simulink model "HEV_Simu_V1_1_RT"  (R2018a)
settings: Solver=ode23s  StartTime=0.0  StopTime=660  FixedStep=0.001  EnableMultiTasking=on
PreLoadFcn:
  | HevSimuVccWs_V1_PreLoad
StartFcn:
  | tic
StopFcn:
  | toc
  | disp(['実時間の' num2str(max(tout)/toc) '倍速'])
model workspace (MAT data in the model file):
  Var = 0
undefined symbols (not defined in the file or in its folder): canChannel
libraries: canmsglib x55, canlib x35, simulink x2, sldrtlib x1
(part 1 of 4)
Description:
  | Ver1 ：
settings Model: SimulationMode=accelerator  Creator=1442442  LastModifiedBy=E00026
settings SolverCC: MaxOrder=2  ZeroCrossControl=DisableAll
settings DataIOCC: SaveFormat=Array  SaveOutput=off  SignalLogging=off  DSMLogging=off
settings OptimizationCC: ExpressionDepthLimit=2147483647  EfficientMapNaN2IntZero=off  LifeSpan=inf
settings DebuggingCC: AlgebraicLoopMsg=error  UnderspecifiedInitializationDetection=Classic  MergeDetectMultiDrivingBlocksExec=none  FcnCallInpInsideContextMsg=warning  StateNameClashWarn=warning  SFUnexpectedBacktrackingDiag=warning  SFNoUnconditionalDefaultTransitionDiag=warning  SFExecutionAtInitializationDiag=none
settings HardwareCC: ProdBitPerPointer=32  ProdBitPerSizeT=32  ProdBitPerPtrDiffT=32  ProdLargestAtomicFloat=None  ProdIntDivRoundTo=Undefined  ProdEndianess=Unspecified  ProdWordSize=32  ProdHWDeviceType=32-bit Generic  TargetBitPerPointer=64  TargetBitPerSizeT=64  TargetBitPerPtrDiffT=64  TargetLongLongMode=on  TargetIntDivRoundTo=Zero  TargetEndianess=LittleEndian  TargetWordSize=64  TargetHWDeviceType=MATLAB Host  ProdEqTarget=off
settings ModelReferenceCC: PropagateSignalLabelsOutOfModel=off
settings CodeAppCC: MaxIdLength=128
settings GRTTargetCC: TargetLangStandard=C89/C90 (ANSI)  CombineOutputUpdateFcns=off  GRTInterface=on
settings ConfigComp: CovMetricSettings=dw  CovHtmlReporting=on  CovSaveCumulativeToWorkspaceVar=on  CovSaveSingleToWorkspaceVar=on  CovExternalEMLEnable=off  CovSFcnEnable=off
settings SimscapeCC: SimscapeNormalizeSystem=off  SimscapeLogSimulationStatistics=on  SimscapeLogOpenViewer=on  SimscapeLogLimitData=off

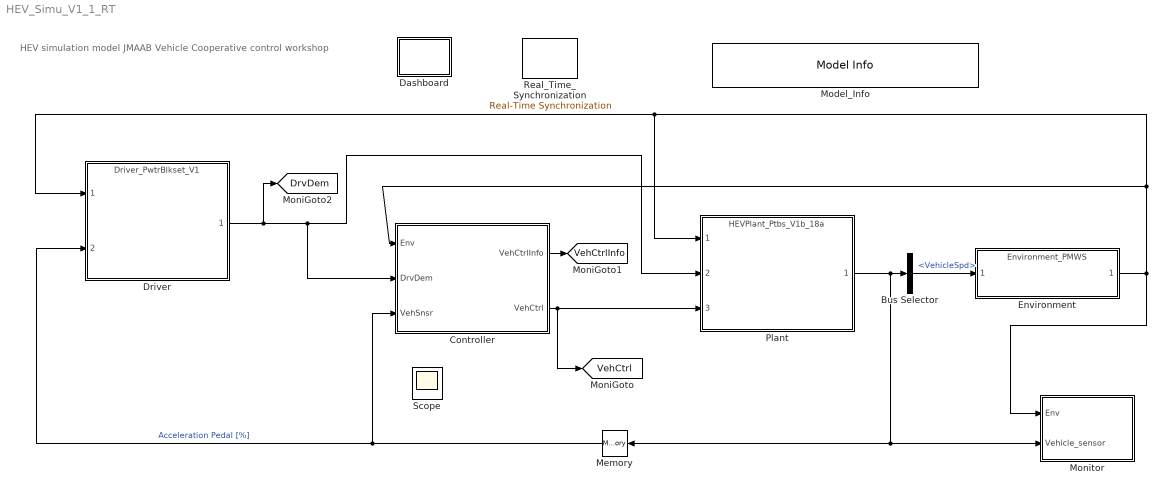
== system HEV_Simu_V1_1_RT ==
  note: HEV simulation model
      | JMAAB Vehicle Cooperative control workshop
  Bus Selector : BusSelector  OutputSignals=Brake_sensor.VehicleSpd
  Controller : Subsystem  Variant=on  PropagateVariantConditions=on
  Dashboard : Subsystem
  Driver : ModelReference  ModelNameDialog=Driver_PwtrBlkset_V1.slx  SimulationMode=Normal  ModelReferenceVersion=1.1301
  Environment : ModelReference  ModelNameDialog=Environment_PMWS.slx  SimulationMode=Normal  ModelReferenceVersion=1.1285
  Memory : Memory
  Model_Info : simulink/Model-Wide Utilities/Model Info  Frame=on  DisplayStringWithTags=|  HorizontalTextAlignment=Left  LeftAlignmentValue=0.02
      | Version  %<ModelVersion>
      | LastModifided by %<LastModifiedBy>  Date %<LastModificationDate>
      | Description  %<Description>
  Monitor : Subsystem
  Plant : ModelReference  ModelNameDialog=HEVPlant_Ptbs_V1b_18a.slx  SimulationMode=Normal  ModelReferenceVersion=1.1342
  Real_Time_Synchronization : sldrtlib/Real-Time Synchronization  SampleTime=0.01  MaxMissedTicks=100  ShowMissedTicks=off  YieldWhenWaiting=off
      settings: AttributesFormatString=<MaxMissedTicks = %<MaxMissedTicks>>
  Scope : Scope
  tag scope: DrvDem=global, VehCtrl=global, VehCtrlInfo=global
  wires:
  Bus Selector/1 -> Environment/1  "<VehicleSpd>"
  Memory/1 -> Driver/2, Controller/3(VehSnsr)  "Acceleration Pedal [%]"
  Plant/1 -> Monitor/2(Vehicle_sensor), Memory/1, Bus Selector/1
  Driver/1 -> Controller/2("DrvDem "), Plant/2, [DrvDem]
  Environment/1 -> Plant/1, Driver/1, Controller/1("Env "), Monitor/1(Env)
  Controller/1(" VehCtrlInfo") -> [VehCtrlInfo]
  Controller/2(" VehCtrl") -> Plant/3, [VehCtrl]

== system HEV_Simu_V1_1_RT/Controller ==
  "Env " : Inport
  "DrvDem " : Inport  Port=2
  VehSnsr : Inport  Port=3
  CtrlStrct_SmplCAN.slx : ModelReference  ModelNameDialog=CtrlStrct_SmplCAN.slx  SimulationMode=Normal  VariantControl=VarObj_CtrlStruct_CAN_Simpl  ModelReferenceVersion=0.1.90
  CtrlStrct_SmplCAN_Intg.slx : ModelReference  ModelNameDialog=CtrlStrct_SmplCAN_Intg.slx  SimulationMode=Normal  VariantControl=(default)  ModelReferenceVersion=0.1.68
  CtrlStrct_SmplCAN_TW.slx : ModelReference  ModelNameDialog=CtrlStrct_SmplCAN_TW.slx  SimulationMode=Normal  VariantControl=VarObj_CtrlStruct_CAN_Simpl_TW  ModelReferenceVersion=0.1.89
  CtrlStrct_VNT_Level_1 : ModelReference  ModelNameDialog=CtrlStrct_VNT_Level1_TW.slx  SimulationMode=Normal  VariantControl=VarObj_CtrlStruct_CAN_VNT_Level_1  ModelReferenceVersion=0.1.98
  CtrlStrct_VNT_Level_2 : Subsystem  TreatAsAtomicUnit=on  VariantControl=VarObj_CtrlStruct_CAN_VNT_Level_2
  " VehCtrlInfo" : Outport
  " VehCtrl" : Outport  Port=2

== system HEV_Simu_V1_1_RT/Dashboard ==
  note: Battery SOC
  note: Brake Pedal
  note: Accel Pedal
  note: Engine Speed
  note: Vehicle Speed
  note: Engine Torque Dem
  note: Clutch Dem
  note: Motor Torque Dem
  Dashboard Scope : Subsystem  DialogController=hmiCreateDDGDialog  IsWebBlock=on  mask(MWDashboardBlock){webBlockId=ed88d156-d389-420b-ac55-88fe2db30599, webBlockType=sdiscope, ShowInitialText=on, HMISrcModelName=HEV_Simu_V1_1_RT}
      mask prompts: webBlockId "WebBlock Id"; webBlockType "WebBlock Type"; HMISrcModelName "Source Model"
      mask help: SimulinkHMI:dialogs:HMIScopeDialogDesc
      mask Help: helpview([docroot '/mapfiles/simulink.map'], 'hmi_scope')
      mask Display:
      | if strcmp(get_param(bdroot(gcb),'BlockDiagramType'), 'library')
      |     image([(matlabroot) '/toolbox/simulink/hmi/icons/DashboardScope.png']);
      | end
  Gauge : Subsystem  DialogController=hmiCreateDDGDialog  IsWebBlock=on  mask(MWDashboardBlock){webBlockId=63f936d2-1b71-4121-bdb3-6f8d7f4bf67f, webBlockType=circulargauge, ShowInLibBrowser=on, ShowInitialText=on, HMISrcModelName=HEV_Simu_V1_1_RT}
      mask prompts: webBlockId "WebBlock Id"; webBlockType "WebBlock Type"; HMISrcModelName "Source Model"
      mask help: SimulinkHMI:dialogs:CircularGaugeDialogDesc
      mask Help: helpview([docroot '/mapfiles/simulink.map'], 'hmi_gauge')
      mask Display:
      | if strcmp(get_param(bdroot(gcb),'BlockDiagramType'), 'library')
      |     image([(matlabroot) '/toolbox/simulink/hmi/icons/CircularGauge.png']);
      | end
  Gauge1 : Subsystem  DialogController=hmiCreateDDGDialog  IsWebBlock=on  mask(MWDashboardBlock){webBlockId=f9ab9f1f-3ce6-4036-8e0e-91baa74d8dba, webBlockType=circulargauge, ShowInLibBrowser=on, ShowInitialText=on, HMISrcModelName=HEV_Simu_V1_1_RT}
      mask prompts: webBlockId "WebBlock Id"; webBlockType "WebBlock Type"; HMISrcModelName "Source Model"
      mask help: SimulinkHMI:dialogs:CircularGaugeDialogDesc
      mask Help: helpview([docroot '/mapfiles/simulink.map'], 'hmi_gauge')
      mask Display:
      | if strcmp(get_param(bdroot(gcb),'BlockDiagramType'), 'library')
      |     image([(matlabroot) '/toolbox/simulink/hmi/icons/CircularGauge.png']);
      | end
  Linear Gauge : Subsystem  DialogController=hmiCreateDDGDialog  IsWebBlock=on  mask(MWDashboardBlock){webBlockId=d39eeb4b-9fab-4e2b-bb63-54dd45bd1f7c, webBlockType=lineargauge, ShowInLibBrowser=on, ShowInitialText=on, HMISrcModelName=HEV_Simu_V1_1_RT}
      mask prompts: webBlockId "WebBlock Id"; webBlockType "WebBlock Type"; HMISrcModelName "Source Model"
      mask help: SimulinkHMI:dialogs:LinearGaugeDialogDesc
      mask Help: helpview([docroot '/mapfiles/simulink.map'], 'hmi_linear_gauge')
      mask Display:
      | if strcmp(get_param(bdroot(gcb),'BlockDiagramType'), 'library')
      |     image([(matlabroot) '/toolbox/simulink/hmi/icons/LinearGauge.png']);
      | end
  Linear Gauge1 : Subsystem  DialogController=hmiCreateDDGDialog  IsWebBlock=on  mask(MWDashboardBlock){webBlockId=fb227460-5497-40ec-922f-134b3e225288, webBlockType=lineargauge, ShowInLibBrowser=on, ShowInitialText=on, HMISrcModelName=HEV_Simu_V1_1_RT}
      mask prompts: webBlockId "WebBlock Id"; webBlockType "WebBlock Type"; HMISrcModelName "Source Model"
      mask help: SimulinkHMI:dialogs:LinearGaugeDialogDesc
      mask Help: helpview([docroot '/mapfiles/simulink.map'], 'hmi_linear_gauge')
      mask Display:
      | if strcmp(get_param(bdroot(gcb),'BlockDiagramType'), 'library')
      |     image([(matlabroot) '/toolbox/simulink/hmi/icons/LinearGauge.png']);
      | end
  Linear Gauge2 : Subsystem  DialogController=hmiCreateDDGDialog  IsWebBlock=on  mask(MWDashboardBlock){webBlockId=1d5b4a74-8e32-404d-8aff-08484f192aeb, webBlockType=lineargauge, ShowInLibBrowser=on, ShowInitialText=on, HMISrcModelName=HEV_Simu_V1_1_RT}
      mask prompts: webBlockId "WebBlock Id"; webBlockType "WebBlock Type"; HMISrcModelName "Source Model"
      mask help: SimulinkHMI:dialogs:LinearGaugeDialogDesc
      mask Help: helpview([docroot '/mapfiles/simulink.map'], 'hmi_linear_gauge')
      mask Display:
      | if strcmp(get_param(bdroot(gcb),'BlockDiagramType'), 'library')
      |     image([(matlabroot) '/toolbox/simulink/hmi/icons/LinearGauge.png']);
      | end
  Linear Gauge3 : Subsystem  DialogController=hmiCreateDDGDialog  IsWebBlock=on  mask(MWDashboardBlock){webBlockId=8d479cc7-cf22-4f0e-9a8d-8e93dc3b7c1a, webBlockType=lineargauge, ShowInLibBrowser=on, ShowInitialText=on, HMISrcModelName=HEV_Simu_V1_1_RT}
      mask prompts: webBlockId "WebBlock Id"; webBlockType "WebBlock Type"; HMISrcModelName "Source Model"
      mask help: SimulinkHMI:dialogs:LinearGaugeDialogDesc
      mask Help: helpview([docroot '/mapfiles/simulink.map'], 'hmi_linear_gauge')
      mask Display:
      | if strcmp(get_param(bdroot(gcb),'BlockDiagramType'), 'library')
      |     image([(matlabroot) '/toolbox/simulink/hmi/icons/LinearGauge.png']);
      | end
  Linear Gauge4 : Subsystem  DialogController=hmiCreateDDGDialog  IsWebBlock=on  mask(MWDashboardBlock){webBlockId=595c5480-ce82-49fb-a87f-a471381cfd80, webBlockType=lineargauge, ShowInLibBrowser=on, ShowInitialText=on, HMISrcModelName=HEV_Simu_V1_1_RT}
      mask prompts: webBlockId "WebBlock Id"; webBlockType "WebBlock Type"; HMISrcModelName "Source Model"
      mask help: SimulinkHMI:dialogs:LinearGaugeDialogDesc
      mask Help: helpview([docroot '/mapfiles/simulink.map'], 'hmi_linear_gauge')
      mask Display:
      | if strcmp(get_param(bdroot(gcb),'BlockDiagramType'), 'library')
      |     image([(matlabroot) '/toolbox/simulink/hmi/icons/LinearGauge.png']);
      | end
  Linear Gauge5 : Subsystem  DialogController=hmiCreateDDGDialog  IsWebBlock=on  mask(MWDashboardBlock){webBlockId=43b93f51-ee21-4470-88be-b6fb93d81e08, webBlockType=lineargauge, ShowInLibBrowser=on, ShowInitialText=on, HMISrcModelName=HEV_Simu_V1_1_RT}
      mask prompts: webBlockId "WebBlock Id"; webBlockType "WebBlock Type"; HMISrcModelName "Source Model"
      mask help: SimulinkHMI:dialogs:LinearGaugeDialogDesc
      mask Help: helpview([docroot '/mapfiles/simulink.map'], 'hmi_linear_gauge')
      mask Display:
      | if strcmp(get_param(bdroot(gcb),'BlockDiagramType'), 'library')
      |     image([(matlabroot) '/toolbox/simulink/hmi/icons/LinearGauge.png']);
      | end

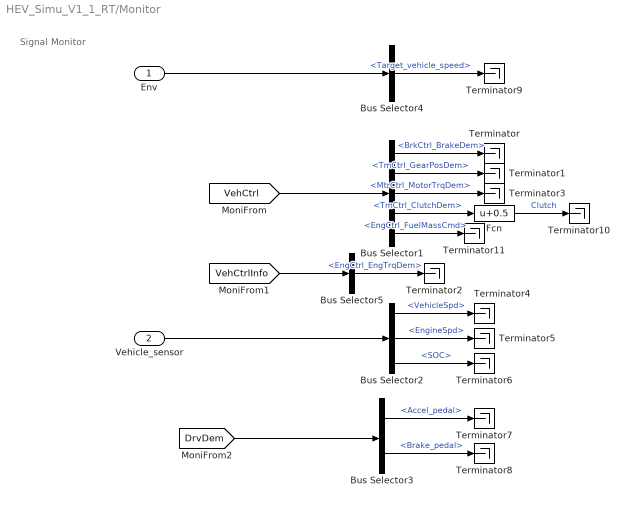
== system HEV_Simu_V1_1_RT/Monitor ==
  note: Signal Monitor
  Env : Inport
  Vehicle_sensor : Inport  Port=2
  Bus Selector1 : BusSelector  OutputSignals=BrakeCtrl.BrkCtrl_BrakeDem,TransmCtrl.TmCtrl_GearPosDem,MotorCtrl.MtrCtrl_MotorTrqDem,TransmCtrl.TmCtrl_ClutchDem,EngineCtrl.EngCtrl_FuelMassCmd
  Bus Selector2 : BusSelector  OutputSignals=Brake_sensor.VehicleSpd,Engine_sensor.EngineSpd,Battery_sensor.SOC
  Bus Selector3 : BusSelector  OutputSignals=Accel_pedal,Brake_pedal
  Bus Selector4 : BusSelector  OutputSignals=Target_vehicle_speed
  Bus Selector5 : BusSelector  OutputSignals=EngineCtrl_Info.EngCtrl_EngTrqDem
  Fcn : Fcn  Expr=u+0.5
  Terminator{,1..11} (12 alike) : Terminator
  wires:
  [VehCtrl] -> Bus Selector1/1
  Vehicle_sensor/1 -> Bus Selector2/1
  Bus Selector1/2 -> Terminator1/1  "<TmCtrl_GearPosDem>"
  Bus Selector1/3 -> Terminator3/1  "<MtrCtrl_MotorTrqDem>"
  Bus Selector2/1 -> Terminator4/1  "<VehicleSpd>"
  Bus Selector2/2 -> Terminator5/1  "<EngineSpd>"
  Bus Selector2/3 -> Terminator6/1  "<SOC>"
  Bus Selector1/1 -> Terminator/1  "<BrkCtrl_BrakeDem>"
  [DrvDem] -> Bus Selector3/1
  Bus Selector3/1 -> Terminator7/1  "<Accel_pedal>"
  Bus Selector3/2 -> Terminator8/1  "<Brake_pedal>"
  Env/1 -> Bus Selector4/1
  Bus Selector4/1 -> Terminator9/1  "<Target_vehicle_speed>"
  [VehCtrlInfo] -> Bus Selector5/1
  Bus Selector5/1 -> Terminator2/1  "<EngCtrl_EngTrqDem>"
  Bus Selector1/4 -> Fcn/1  "<TmCtrl_ClutchDem>"
  Fcn/1 -> Terminator10/1  "Clutch"
  Bus Selector1/5 -> Terminator11/1  "<EngCtrl_FuelMassCmd>"

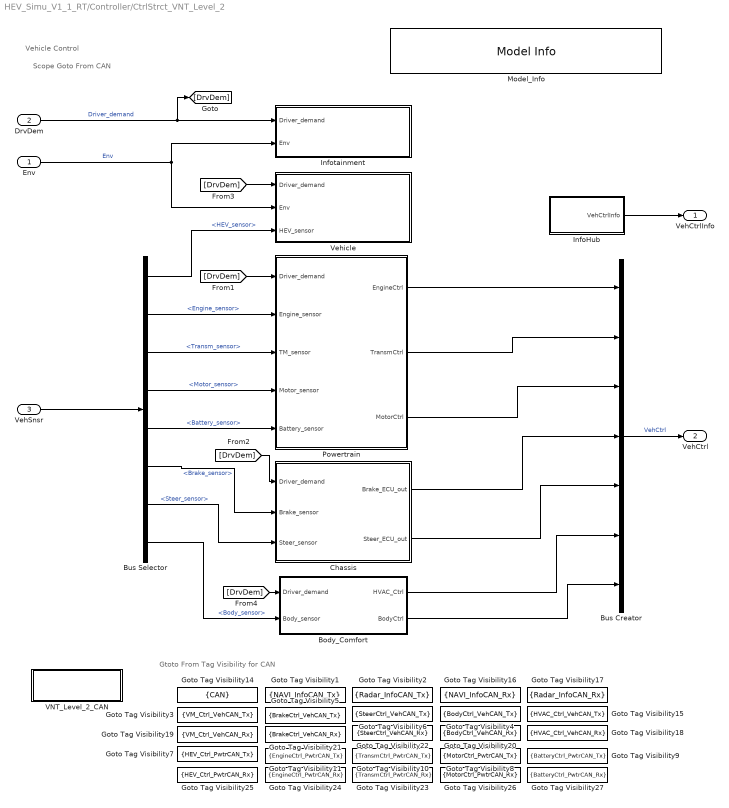
== system HEV_Simu_V1_1_RT/Controller/CtrlStrct_VNT_Level_2 ==
  note: Vehicle Control
  note: Gtoto From Tag Visibility for CAN
  note: Scope Goto From CAN
  Env : Inport  OutDataTypeStr=Bus: Environment_Bus
      settings: AttributesFormatString=<%<OutDataTypeStr>>
  DrvDem : Inport  Port=2  OutDataTypeStr=Bus: Driver_demand_Bus
      settings: AttributesFormatString=%<OutDataTypeStr>
  VehSnsr : Inport  Port=3  OutDataTypeStr=Bus: Vehicle_sensor_Bus
      settings: AttributesFormatString=<%<OutDataTypeStr>>
  Body_Comfort : Subsystem
  Bus Creator : BusCreator  Inputs=7  OutDataTypeStr=Bus: Ctrl_intg_Bus
      settings: AttributesFormatString=%<OutDataTypeStr>
  Bus Selector : BusSelector  OutputSignals=HEV_sensor,Engine_sensor,Transm_sensor,Motor_sensor,Battery_sensor,Brake_sensor,Steer_sensor,Body_sensor
  Chassis : Subsystem
  Goto Tag Visibility1 : GotoTagVisibility  GotoTag=NAVI_InfoCAN_Tx
  Goto Tag Visibility10 : GotoTagVisibility  GotoTag=TransmCtrl_PwtrCAN_Tx
  Goto Tag Visibility11 : GotoTagVisibility  GotoTag=EngineCtrl_PwtrCAN_Tx
  Goto Tag Visibility14 : GotoTagVisibility  GotoTag=CAN
  Goto Tag Visibility15 : GotoTagVisibility  GotoTag=HVAC_Ctrl_VehCAN_Tx
  Goto Tag Visibility16 : GotoTagVisibility  GotoTag=NAVI_InfoCAN_Rx
  Goto Tag Visibility17 : GotoTagVisibility  GotoTag=Radar_InfoCAN_Rx
  Goto Tag Visibility18 : GotoTagVisibility  GotoTag=HVAC_Ctrl_VehCAN_Rx
  Goto Tag Visibility19 : GotoTagVisibility  GotoTag=VM_Ctrl_VehCAN_Rx
  Goto Tag Visibility2 : GotoTagVisibility  GotoTag=Radar_InfoCAN_Tx
  Goto Tag Visibility20 : GotoTagVisibility  GotoTag=BodyCtrl_VehCAN_Rx
  Goto Tag Visibility21 : GotoTagVisibility  GotoTag=BrakeCtrl_VehCAN_Rx
  Goto Tag Visibility22 : GotoTagVisibility  GotoTag=SteerCtrl_VehCAN_Rx
  Goto Tag Visibility23 : GotoTagVisibility  GotoTag=TransmCtrl_PwtrCAN_Rx
  Goto Tag Visibility24 : GotoTagVisibility  GotoTag=EngineCtrl_PwtrCAN_Rx
  Goto Tag Visibility25 : GotoTagVisibility  GotoTag=HEV_Ctrl_PwtrCAN_Rx
  Goto Tag Visibility26 : GotoTagVisibility  GotoTag=MotorCtrl_PwtrCAN_Rx
  Goto Tag Visibility27 : GotoTagVisibility  GotoTag=BatteryCtrl_PwtrCAN_Rx
  Goto Tag Visibility3 : GotoTagVisibility  GotoTag=VM_Ctrl_VehCAN_Tx
  Goto Tag Visibility4 : GotoTagVisibility  GotoTag=BodyCtrl_VehCAN_Tx
  Goto Tag Visibility5 : GotoTagVisibility  GotoTag=BrakeCtrl_VehCAN_Tx
  Goto Tag Visibility6 : GotoTagVisibility  GotoTag=SteerCtrl_VehCAN_Tx
  Goto Tag Visibility7 : GotoTagVisibility  GotoTag=HEV_Ctrl_PwtrCAN_Tx
  Goto Tag Visibility8 : GotoTagVisibility  GotoTag=MotorCtrl_PwtrCAN_Tx
  Goto Tag Visibility9 : GotoTagVisibility  GotoTag=BatteryCtrl_PwtrCAN_Tx
  InfoHub : Subsystem
  Infotainment : Subsystem
  Model_Info : simulink/Model-Wide Utilities/Model Info  Frame=on  DisplayStringWithTags=|  HorizontalTextAlignment=Left  LeftAlignmentValue=0.02
      | Version  %<ModelVersion>
      | LastModifided by %<LastModifiedBy>  Date %<LastModificationDate>
      | Description  %<Description>
  Powertrain : Subsystem
  VNT_Level_2_CAN : Subsystem  VariantControl=VarObj_CanType_VNT_simu
  Vehicle : Subsystem
  VehCtrlInfo : Outport  OutDataTypeStr=Bus: IntgCtrl_Info_Bus
      settings: AttributesFormatString=<%<OutDataTypeStr>>
  VehCtrl : Outport  Port=2  OutDataTypeStr=Bus: Ctrl_intg_Bus
      settings: AttributesFormatString=<%<OutDataTypeStr>>
  wires:
  Chassis/2(Steer_ECU_out) -> Bus Creator/5
  Powertrain/3(MotorCtrl) -> Bus Creator/3
  Env/1 -> Infotainment/2(Env), Vehicle/2(Env)  "Env"
  Bus Selector/3 -> Powertrain/3(TM_sensor)  "<Transm_sensor>"
  InfoHub/1(VehCtrlInfo) -> VehCtrlInfo/1
  Powertrain/2(TransmCtrl) -> Bus Creator/2
  Bus Selector/6 -> Chassis/2(Brake_sensor)  "<Brake_sensor>"
  [DrvDem] -> Chassis/1(Driver_demand)
  Bus Selector/2 -> Powertrain/2(Engine_sensor)  "<Engine_sensor>"
  Bus Selector/7 -> Chassis/3(Steer_sensor)  "<Steer_sensor>"
  Body_Comfort/2(BodyCtrl) -> Bus Creator/7
  VehSnsr/1 -> Bus Selector/1
  [DrvDem] -> Body_Comfort/1(Driver_demand)
  Bus Selector/4 -> Powertrain/4(Motor_sensor)  "<Motor_sensor>"
  Bus Selector/8 -> Body_Comfort/2(Body_sensor)  "<Body_sensor>"
  Bus Selector/1 -> Vehicle/3(HEV_sensor)  "<HEV_sensor>"
  Powertrain/1(EngineCtrl) -> Bus Creator/1
  Body_Comfort/1(HVAC_Ctrl) -> Bus Creator/6
  Bus Creator/1 -> VehCtrl/1  "VehCtrl"
  [DrvDem] -> Vehicle/1(Driver_demand)
  Bus Selector/5 -> Powertrain/5(Battery_sensor)  "<Battery_sensor>"
  Chassis/1(Brake_ECU_out) -> Bus Creator/4
  [DrvDem] -> Powertrain/1(Driver_demand)
  DrvDem/1 -> Infotainment/1(Driver_demand), [DrvDem]  "Driver_demand"

== system HEV_Simu_V1_1_RT/Dashboard/Dashboard Scope ==

== system HEV_Simu_V1_1_RT/Dashboard/Gauge ==

== system HEV_Simu_V1_1_RT/Dashboard/Gauge1 ==

== system HEV_Simu_V1_1_RT/Dashboard/Linear Gauge ==

== system HEV_Simu_V1_1_RT/Dashboard/Linear Gauge1 ==

== system HEV_Simu_V1_1_RT/Dashboard/Linear Gauge2 ==

== system HEV_Simu_V1_1_RT/Dashboard/Linear Gauge3 ==

== system HEV_Simu_V1_1_RT/Dashboard/Linear Gauge4 ==

== system HEV_Simu_V1_1_RT/Dashboard/Linear Gauge5 ==

== system HEV_Simu_V1_1_RT/Controller/CtrlStrct_VNT_Level_2/Body_Comfort ==
  note: Body Control
  Driver_demand : Inport
  Body_sensor : Inport  Port=2
  Body_Control : Subsystem
  HVAC_Control : Subsystem
  HVAC_Ctrl : Outport
  BodyCtrl : Outport  Port=2
  wires:
  HVAC_Control/1(HVAC_Ctrl) -> HVAC_Ctrl/1
  Body_sensor/1 -> Body_Control/2(Body_sensor), HVAC_Control/2(Body_sensor)
  Driver_demand/1 -> Body_Control/1(Driver_demand), HVAC_Control/1(Driver_demand)
  Body_Control/1(BodyCtrl) -> BodyCtrl/1

== system HEV_Simu_V1_1_RT/Controller/CtrlStrct_VNT_Level_2/Chassis ==
  note: Chassis Control
  Driver_demand : Inport
  Brake_sensor : Inport  Port=2
  Steer_sensor : Inport  Port=3
  Brake_Control : Subsystem
  Steer_Control : Subsystem
  Brake_ECU_out : Outport
  Steer_ECU_out : Outport  Port=2
  wires:
  Steer_sensor/1 -> Steer_Control/2(Steer_sensor)
  Steer_Control/1(SteerCtrl) -> Steer_ECU_out/1
  Brake_sensor/1 -> Brake_Control/2(Brake_sensor)
  Brake_Control/1(BrakeCtrl) -> Brake_ECU_out/1
  Driver_demand/1 -> Steer_Control/1(Driver_demand), Brake_Control/1(Driver_demand)

== system HEV_Simu_V1_1_RT/Controller/CtrlStrct_VNT_Level_2/InfoHub ==
  Bus Creator1 : BusCreator  Inputs=2
  Bus Selector : BusSelector  OutputSignals=VehCAN.BrakeCtrl_VehCAN_Tx_0CFF600B,PwtrCAN.EngineCtrl_PwtrCAN_Tx_0CFF3000
  CAN Unpack10 : canmsglib/CAN Unpack  CANdbFile=C:\Users\aa781680\OneDrive - YanmarGlobal\MainStrage\04_MATLAB\JMAAB_CoopCon\CoopConModel\20180726_18a_ymr\Project\CANDB\HEV_CANDB.dbc  MsgList=EngineCtrl_PwtrCAN_Tx  MsgName=EngineCtrl_PwtrCAN_Tx  MsgIDType=Extended (29-bit identifier)  MsgIdentifier=218050560  MsgLength=8  SignalInfo=EngCtrl_Engine_speed$0$16$1$2$1$0$1.250000e-01$0$0$8192$#EngCtrl_Engine_torque_actual$16$16$1$1$1$0$1.562500e-02$0$-300$300$#  NSignals=2  IDPort=off  TimestampPort=off  ErrorPort=off  RemotePort=off  LengthPort=off  StatusPort=off  StartBits=str2num('[int32(0);int32(16)]')  SignalSizes=str2num('[int32(16);int32(16)]')  ByteOrders=str2num('[int32(1);int32(1)]')  DataTypes=str2num('[int32(2);int32(1)]')  MultiplexTypes=str2num('[int32(1);int32(1)]')  MultiplexValues=str2num('[double(0);double(0)]')  Factors=str2num('[double(1.250000e-01);double(1.562500e-02)]')  Offsets=str2num('[double(0);double(0)]')  Minimums=str2num('[double(0);double(-300)]')  Maximums=str2num('[double(8192);double(300)]')  ApplyMinMax=off
      settings: SourceProductName=Simulink Real-Time  SourceProductBaseCode=XP  DataFormat=CANdb specified signals
  CAN Unpack3 : canmsglib/CAN Unpack  CANdbFile=C:\Users\aa781680\OneDrive - YanmarGlobal\MainStrage\04_MATLAB\JMAAB_CoopCon\CoopConModel\20180726_18a_ymr\Project\CANDB\HEV_CANDB.dbc  MsgList=BrakeCtrl_VehCAN_Tx  MsgName=BrakeCtrl_VehCAN_Tx  MsgIDType=Extended (29-bit identifier)  MsgIdentifier=218062859  MsgLength=8  SignalInfo=BrkCtrl_Regen_brake_torque_reque$16$16$1$1$1$0$1.000000e-02$0$-300$300$#BrkCtrl_Vehicle_speed$0$16$1$2$1$0$1.000000e-01$0$0$180$#  NSignals=2  IDPort=off  TimestampPort=off  ErrorPort=off  RemotePort=off  LengthPort=off  StatusPort=off  StartBits=str2num('[int32(16);int32(0)]')  SignalSizes=str2num('[int32(16);int32(16)]')  ByteOrders=str2num('[int32(1);int32(1)]')  DataTypes=str2num('[int32(1);int32(2)]')  MultiplexTypes=str2num('[int32(1);int32(1)]')  MultiplexValues=str2num('[double(0);double(0)]')  Factors=str2num('[double(1.000000e-02);double(1.000000e-01)]')  Offsets=str2num('[double(0);double(0)]')  Minimums=str2num('[double(-300);double(0)]')  Maximums=str2num('[double(300);double(180)]')  ApplyMinMax=off
      settings: SourceProductName=Simulink Real-Time  SourceProductBaseCode=XP  DataFormat=CANdb specified signals
  Terminator{1..4} (4 alike) : Terminator
  VehCtrlInfo : Outport
  wires:
  [CAN] -> Bus Selector/1
  Bus Creator1/1 -> VehCtrlInfo/1  "VehCtrlInfo"
  [Engine_ECU_Info] -> Bus Creator1/2
  [HEV_ECU_Info] -> Bus Creator1/1
  CAN Unpack10/2 -> Terminator1/1
  Bus Selector/1 -> CAN Unpack10/1  "<BrakeCtrl_VehCAN_Tx_0CFF600B>"
  CAN Unpack3/1 -> Terminator2/1
  Bus Selector/2 -> CAN Unpack3/1  "<EngineCtrl_PwtrCAN_Tx_0CFF3000>"
  CAN Unpack10/1 -> Terminator3/1  "EngCtrl_Engine_speed"
  CAN Unpack3/2 -> Terminator4/1  "BrkCtrl_Vehicle_speed"

== system HEV_Simu_V1_1_RT/Controller/CtrlStrct_VNT_Level_2/Infotainment ==
  note: Infotainment
  Driver_demand : Inport
  Env : Inport  Port=2
  Navigation : Subsystem
  Radar_Detection : Subsystem
  wires:
  Driver_demand/1 -> Navigation/1(Driver_demand), Radar_Detection/1(Driver_demand)
  Env/1 -> Radar_Detection/2(Env), Navigation/2(Env)

== system HEV_Simu_V1_1_RT/Controller/CtrlStrct_VNT_Level_2/Powertrain ==
  note: Powertrain Control
  Driver_demand : Inport
  Engine_sensor : Inport  Port=2
  TM_sensor : Inport  Port=3
  Motor_sensor : Inport  Port=4
  Battery_sensor : Inport  Port=5
  Battery_Control : Subsystem
  Engine_Control : Subsystem
  Motor_Control : Subsystem
  Transm_Control : Subsystem
  EngineCtrl : Outport
  TransmCtrl : Outport  Port=2
  MotorCtrl : Outport  Port=3
  wires:
  TM_sensor/1 -> Transm_Control/2(TM_sensor)
  Transm_Control/1(TransmCtrl) -> TransmCtrl/1
  Engine_sensor/1 -> Engine_Control/2(Engine_sensor)
  Engine_Control/1(EngineCtrl) -> EngineCtrl/1
  Battery_sensor/1 -> Battery_Control/1(Battery_sensor)
  Motor_sensor/1 -> Motor_Control/1(Motor_sensor)
  Motor_Control/1(MotorCtrl) -> MotorCtrl/1
  Driver_demand/1 -> Engine_Control/1(Driver_demand), Transm_Control/1(Driver_demand)

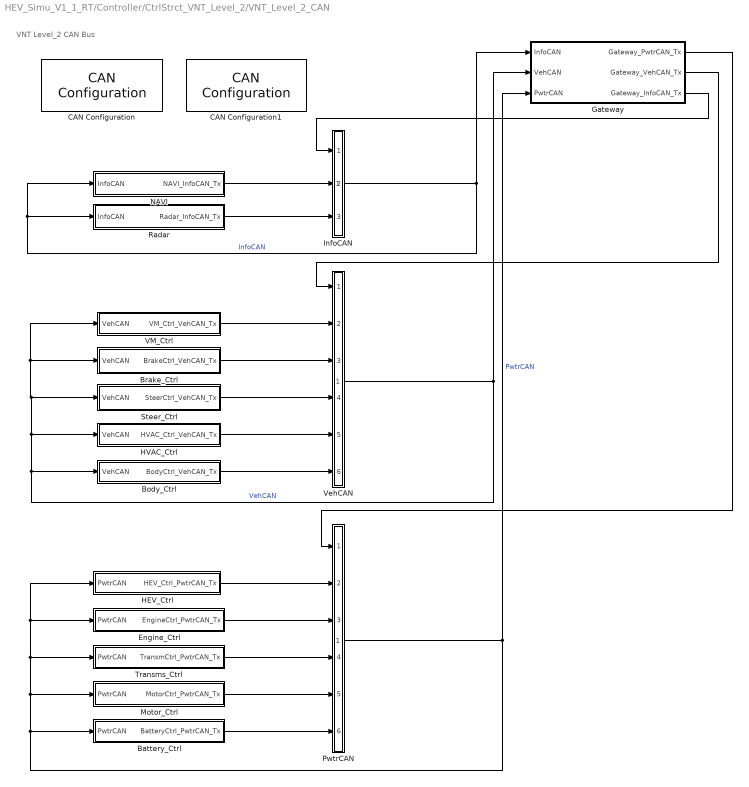
== system HEV_Simu_V1_1_RT/Controller/CtrlStrct_VNT_Level_2/VNT_Level_2_CAN ==
  note: VNT Level_2 CAN Bus
  Battery_Ctrl : Subsystem
  Body_Ctrl : Subsystem
  Brake_Ctrl : Subsystem
  CAN Configuration : canlib/CAN Configuration  BlockHandle=15943.0026  DeviceMenu=Vector CANcaseXL 1 (Channel 1)  Device=Vector CANcaseXL 1 (Channel 1)  ObjConstructor=canChannel('Vector','CANcaseXL 1',1)  BusSpeed=500000  EnableBitParameters=off  SJW=1  TSEG1=4  TSEG2=3  NSamples=1  AckMode=Normal
      settings: SourceProductName=Vehicle Network Toolbox  SourceProductBaseCode=VN
  CAN Configuration1 : canlib/CAN Configuration  BlockHandle=15944.0026  DeviceMenu=Vector CANcaseXL 1 (Channel 2)  Device=Vector CANcaseXL 1 (Channel 2)  ObjConstructor=canChannel('Vector','CANcaseXL 1',2)  BusSpeed=500000  EnableBitParameters=off  SJW=1  TSEG1=4  TSEG2=3  NSamples=1  AckMode=Normal
      settings: SourceProductName=Vehicle Network Toolbox  SourceProductBaseCode=VN
  Engine_Ctrl : Subsystem
  Gateway : Subsystem
  HEV_Ctrl : Subsystem
  HVAC_Ctrl : Subsystem
  InfoCAN : Subsystem
  Motor_Ctrl : Subsystem
  NAVI : Subsystem
  PwtrCAN : Subsystem
  Radar : Subsystem
  Steer_Ctrl : Subsystem
  Transms_Ctrl : Subsystem
  VM_Ctrl : Subsystem
  VehCAN : Subsystem
  wires:
  Radar/1(Radar_InfoCAN_Tx) -> InfoCAN/3(Radar_InfoCAN_Tx)
  NAVI/1(NAVI_InfoCAN_Tx) -> InfoCAN/2(NAVI_InfoCAN_Tx)
  VM_Ctrl/1(VM_Ctrl_VehCAN_Tx) -> VehCAN/2(VM_Ctrl_VehCAN_Tx)
  Brake_Ctrl/1(BrakeCtrl_VehCAN_Tx) -> VehCAN/3(BrakeCtrl_VehCAN_Tx)
  Steer_Ctrl/1(SteerCtrl_VehCAN_Tx) -> VehCAN/4(SteerCtrl_VehCAN_Tx)
  HVAC_Ctrl/1(HVAC_Ctrl_VehCAN_Tx) -> VehCAN/5(HVAC_Ctrl_VehCAN_Tx)
  Body_Ctrl/1(BodyCtrl_VehCAN_Tx) -> VehCAN/6(BodyCtrl_VehCAN_Tx)
  Battery_Ctrl/1(BatteryCtrl_PwtrCAN_Tx) -> PwtrCAN/6(BatteryCtrl_PwtrCAN_Tx)
  Transms_Ctrl/1(TransmCtrl_PwtrCAN_Tx) -> PwtrCAN/4(TransmCtrl_PwtrCAN_Tx)
  Motor_Ctrl/1(MotorCtrl_PwtrCAN_Tx) -> PwtrCAN/5(MotorCtrl_PwtrCAN_Tx)
  Gateway/3(Gateway_InfoCAN_Tx) -> InfoCAN/1(Gateway_InfoCAN)
  InfoCAN/1(InfoCAN) -> NAVI/1(InfoCAN), Radar/1(InfoCAN), Gateway/1(InfoCAN)  "InfoCAN"
  Gateway/2(Gateway_VehCAN_Tx) -> VehCAN/1(Gateway_VehCAN_Tx)
  Gateway/1(Gateway_PwtrCAN_Tx) -> PwtrCAN/1(Gateway_PwtrCAN_Tx)
  PwtrCAN/1(PwtrCAN) -> Battery_Ctrl/1(PwtrCAN), HEV_Ctrl/1(PwtrCAN), Engine_Ctrl/1(PwtrCAN), Transms_Ctrl/1(PwtrCAN), Motor_Ctrl/1(PwtrCAN), Gateway/3(PwtrCAN)  "PwtrCAN"
  VehCAN/1(VehCAN) -> Gateway/2(VehCAN), HVAC_Ctrl/1(VehCAN), Brake_Ctrl/1(VehCAN), VM_Ctrl/1(VehCAN), Steer_Ctrl/1(VehCAN), Body_Ctrl/1(VehCAN)  "VehCAN"
  HEV_Ctrl/1(HEV_Ctrl_PwtrCAN_Tx) -> PwtrCAN/2(HEV_Ctrl_PwtrCAN_Tx)
  Engine_Ctrl/1(EngineCtrl_PwtrCAN_Tx) -> PwtrCAN/3(EngineCtrl_PwtrCAN_Tx)

== system HEV_Simu_V1_1_RT/Controller/CtrlStrct_VNT_Level_2/Vehicle ==
  note: Vehicle Integrated Control
  Driver_demand : Inport
  Env : Inport  Port=2
  HEV_sensor : Inport  Port=3
  HEV_Control : Subsystem
  Vehicle_Motion_Control : Subsystem
  wires:
  HEV_sensor/1 -> HEV_Control/2(HEV_sensor)
  Driver_demand/1 -> HEV_Control/1(Driver_demand)
  Env/1 -> Vehicle_Motion_Control/1(Env)

== system HEV_Simu_V1_1_RT/Controller/CtrlStrct_VNT_Level_2/Body_Comfort/Body_Control ==
  note: Body Control
  Driver_demand : Inport
  Body_sensor : Inport  Port=2
  BodyControlModule : ModelReference  ModelNameDialog=BodyCtrl_V1_1.slx  SimulationMode=Normal  ModelReferenceVersion=0.1.16
  Rate Transition1 : RateTransition  Deterministic=off
      settings: AttributesFormatString=<Deterministic=%<Deterministic>>
  Rate Transition2 : RateTransition  Deterministic=off
      settings: AttributesFormatString=<Deterministic=%<Deterministic>>
  Rate Transition4 : RateTransition  Deterministic=off
      settings: AttributesFormatString=<Deterministic=%<Deterministic>>
  BodyCtrl : Outport
  tag scope: BodyCtrl_VehCAN_Tx=scoped
  wires:
  Rate Transition1/1 -> BodyControlModule/2
  Body_sensor/1 -> Rate Transition1/1
  Rate Transition4/1 -> BodyCtrl/1  "BodyCtrl"
  BodyControlModule/2 -> [BodyCtrl_VehCAN_Tx]  "BodyCtrl_VehCAN_Tx"
  [BodyCtrl_VehCAN_Rx] -> BodyControlModule/3
  BodyControlModule/1 -> Rate Transition4/1
  Rate Transition2/1 -> BodyControlModule/1
  Driver_demand/1 -> Rate Transition2/1

== system HEV_Simu_V1_1_RT/Controller/CtrlStrct_VNT_Level_2/Body_Comfort/HVAC_Control ==
  note: HVAC Control
  Driver_demand : Inport
  Body_sensor : Inport  Port=2
  Aircon_Control : ModelReference  ModelNameDialog=HVAC_Ctrl_V1_1.slx  SimulationMode=Normal  ModelReferenceVersion=0.1.25
  Rate Transition1 : RateTransition  Deterministic=off
      settings: AttributesFormatString=<Deterministic=%<Deterministic>>
  Rate Transition2 : RateTransition  Deterministic=off
      settings: AttributesFormatString=<Deterministic=%<Deterministic>>
  Rate Transition4 : RateTransition  Deterministic=off
      settings: AttributesFormatString=<Deterministic=%<Deterministic>>
  HVAC_Ctrl : Outport
  tag scope: HVAC_Ctrl_VehCAN_Tx=scoped
  wires:
  Driver_demand/1 -> Rate Transition2/1
  Rate Transition2/1 -> Aircon_Control/1
  Aircon_Control/1 -> Rate Transition4/1
  [HVAC_Ctrl_VehCAN_Rx] -> Aircon_Control/3
  Aircon_Control/2 -> [HVAC_Ctrl_VehCAN_Tx]  "HVAC_Ctrl_VehCAN_Tx"
  Rate Transition4/1 -> HVAC_Ctrl/1  "HVAC_Ctrl"
  Body_sensor/1 -> Rate Transition1/1
  Rate Transition1/1 -> Aircon_Control/2

== system HEV_Simu_V1_1_RT/Controller/CtrlStrct_VNT_Level_2/Chassis/Brake_Control ==
  note: Brake Control
  Driver_demand : Inport
  Brake_sensor : Inport  Port=2
  Brake_Control : ModelReference  ModelNameDialog=BrakeCtrl_V1_1.slx  SimulationMode=Normal  ModelReferenceVersion=1.0.23
  Rate Transition1 : RateTransition  Deterministic=off
      settings: AttributesFormatString=<Deterministic=%<Deterministic>>
  Rate Transition2 : RateTransition  Deterministic=off
      settings: AttributesFormatString=<Deterministic=%<Deterministic>>
  Rate Transition4 : RateTransition  Deterministic=off
      settings: AttributesFormatString=<Deterministic=%<Deterministic>>
  Terminator : Terminator
  BrakeCtrl : Outport
  tag scope: BrakeCtrl_VehCAN_Tx=scoped
  wires:
  Brake_Control/2 -> [BrakeCtrl_VehCAN_Tx]  "BrakeCtrl_VehCAN_Tx"
  Brake_Control/1 -> Rate Transition4/1
  Rate Transition4/1 -> BrakeCtrl/1  "BrakeCtrl"
  [BrakeCtrl_VehCAN_Rx] -> Brake_Control/3
  Brake_Control/3 -> Terminator/1
  Brake_sensor/1 -> Rate Transition2/1
  Rate Transition1/1 -> Brake_Control/1
  Driver_demand/1 -> Rate Transition1/1
  Rate Transition2/1 -> Brake_Control/2

== system HEV_Simu_V1_1_RT/Controller/CtrlStrct_VNT_Level_2/Chassis/Steer_Control ==
  note: Steering Control
  Driver_demand : Inport
  Steer_sensor : Inport  Port=2
  Rate Transition3 : RateTransition  Deterministic=off
      settings: AttributesFormatString=<Deterministic=%<Deterministic>>
  Rate Transition4 : RateTransition  Deterministic=off
      settings: AttributesFormatString=<Deterministic=%<Deterministic>>
  Rate Transition5 : RateTransition  Deterministic=off
      settings: AttributesFormatString=<Deterministic=%<Deterministic>>
  Steer_Control : ModelReference  ModelNameDialog=SteerCtrl_V1_1.slx  SimulationMode=Normal  ModelReferenceVersion=0.1.16
  SteerCtrl : Outport
  tag scope: SteerCtrl_VehCAN_Tx=scoped
  wires:
  Steer_Control/2 -> [SteerCtrl_VehCAN_Tx]  "SteerCtrl_VehCAN_Tx"
  Rate Transition5/1 -> SteerCtrl/1  "SteerCtrl"
  Rate Transition3/1 -> Steer_Control/1
  [SteerCtrl_VehCAN_Rx] -> Steer_Control/3
  Steer_sensor/1 -> Rate Transition4/1
  Steer_Control/1 -> Rate Transition5/1
  Driver_demand/1 -> Rate Transition3/1
  Rate Transition4/1 -> Steer_Control/2

== system HEV_Simu_V1_1_RT/Controller/CtrlStrct_VNT_Level_2/Infotainment/Navigation ==
  note: Navigation
  Driver_demand : Inport
  Env : Inport  Port=2
  NAVI : ModelReference  ModelNameDialog=NAVI_V1_1.slx  SimulationMode=Normal  ModelReferenceVersion=0.1.17
  Rate Transition1 : RateTransition  Deterministic=off
      settings: AttributesFormatString=<Deterministic=%<Deterministic>>
  Rate Transition4 : RateTransition  Deterministic=off
      settings: AttributesFormatString=<Deterministic=%<Deterministic>>
  tag scope: NAVI_InfoCAN_Tx=scoped
  wires:
  Rate Transition4/1 -> NAVI/2
  Env/1 -> Rate Transition4/1
  NAVI/1 -> [NAVI_InfoCAN_Tx]  "NAVI_InfoCAN_Tx"
  [NAVI_InfoCAN_Rx] -> NAVI/3
  Driver_demand/1 -> Rate Transition1/1
  Rate Transition1/1 -> NAVI/1

== system HEV_Simu_V1_1_RT/Controller/CtrlStrct_VNT_Level_2/Infotainment/Radar_Detection ==
  note: Radar Detection
  Driver_demand : Inport
  Env : Inport  Port=2
  Radar_Detection : ModelReference  ModelNameDialog=Radar_V1_1.slx  SimulationMode=Normal  ModelReferenceVersion=0.1.17
  Rate Transition1 : RateTransition  Deterministic=off
      settings: AttributesFormatString=<Deterministic=%<Deterministic>>
  Rate Transition4 : RateTransition  Deterministic=off
      settings: AttributesFormatString=<Deterministic=%<Deterministic>>
  tag scope: Radar_InfoCAN_Tx=scoped
  wires:
  Rate Transition4/1 -> Radar_Detection/1
  Driver_demand/1 -> Rate Transition4/1
  Radar_Detection/1 -> [Radar_InfoCAN_Tx]  "Radar_InfoCAN_Tx"
  [Radar_InfoCAN_Rx] -> Radar_Detection/3
  Env/1 -> Rate Transition1/1
  Rate Transition1/1 -> Radar_Detection/2

== system HEV_Simu_V1_1_RT/Controller/CtrlStrct_VNT_Level_2/Powertrain/Battery_Control ==
  note: Battery Control
  Battery_sensor : Inport
  Battery_Control : ModelReference  ModelNameDialog=BatteryCtrl_V1_1.slx  SimulationMode=Normal  ModelReferenceVersion=0.1.22
  Rate Transition1 : RateTransition  Deterministic=off
      settings: AttributesFormatString=<Deterministic=%<Deterministic>>
  tag scope: BatteryCtrl_PwtrCAN_Tx=scoped
  wires:
  Battery_Control/1 -> [BatteryCtrl_PwtrCAN_Tx]  "BatteryCtrl_PwtrCAN_Tx"
  Rate Transition1/1 -> Battery_Control/1
  [BatteryCtrl_PwtrCAN_Rx] -> Battery_Control/2
  Battery_sensor/1 -> Rate Transition1/1

== system HEV_Simu_V1_1_RT/Controller/CtrlStrct_VNT_Level_2/Powertrain/Engine_Control ==
  note: Engine Control
  Driver_demand : Inport
  Engine_sensor : Inport  Port=2
  Engine_Control : Subsystem  Variant=on
  Info_in : Subsystem
  Rate Transition{1..2,5..6} (4 alike) : RateTransition  Deterministic=off
      settings: AttributesFormatString=<Deterministic=%<Deterministic>>
  EngineCtrl : Outport
  tag scope: EngineCtrl_PwtrCAN_Tx=scoped, Engine_ECU_Info=global
  wires:
  Engine_Control/3(" EngineCtrl_Info") -> Rate Transition6/1
  Engine_Control/1(" EngineCtrl") -> Rate Transition5/1
  Info_in/1(Info_in) -> Engine_Control/4("Info_in ")
  [EngineCtrl_PwtrCAN_Rx] -> Engine_Control/3(EngineCtrl_PwtrCAN_Rx)
  Rate Transition2/1 -> Engine_Control/2("Eng_Sns ")
  Rate Transition1/1 -> Engine_Control/1("DrvDem ")
  Engine_Control/2(" EngineCtrl_PwtrCAN_Tx") -> [EngineCtrl_PwtrCAN_Tx]  "EngineCtrl_PwtrCAN_Tx"
  Rate Transition6/1 -> [Engine_ECU_Info]  "EngineCtrl_Info"
  Rate Transition5/1 -> EngineCtrl/1  "EngineCtrl"
  Engine_sensor/1 -> Rate Transition2/1
  Driver_demand/1 -> Rate Transition1/1

== system HEV_Simu_V1_1_RT/Controller/CtrlStrct_VNT_Level_2/Powertrain/Motor_Control ==
  note: Motor Control
  Motor_sensor : Inport
  Motor_Control : ModelReference  ModelNameDialog=MotorCtrl_V1_1.slx  SimulationMode=Normal  ModelReferenceVersion=1.0.21
  Rate Transition1 : RateTransition  Deterministic=off
      settings: AttributesFormatString=<Deterministic=%<Deterministic>>
  Rate Transition3 : RateTransition  Deterministic=off
      settings: AttributesFormatString=<Deterministic=%<Deterministic>>
  Terminator : Terminator
  MotorCtrl : Outport
  tag scope: MotorCtrl_PwtrCAN_Tx=scoped
  wires:
  Motor_Control/2 -> [MotorCtrl_PwtrCAN_Tx]  "MotorCtrl_PwtrCAN_Tx"
  Motor_Control/1 -> Rate Transition3/1
  Rate Transition3/1 -> MotorCtrl/1  "MotorCtrl"
  Motor_Control/3 -> Terminator/1
  Motor_sensor/1 -> Rate Transition1/1
  [MotorCtrl_PwtrCAN_Rx] -> Motor_Control/2
  Rate Transition1/1 -> Motor_Control/1

== system HEV_Simu_V1_1_RT/Controller/CtrlStrct_VNT_Level_2/Powertrain/Transm_Control ==
  note: Transmission Control
  Driver_demand : Inport
  TM_sensor : Inport  Port=2
  Rate Transition3 : RateTransition  Deterministic=off
      settings: AttributesFormatString=<Deterministic=%<Deterministic>>
  Rate Transition4 : RateTransition  Deterministic=off
      settings: AttributesFormatString=<Deterministic=%<Deterministic>>
  Rate Transition5 : RateTransition  Deterministic=off
      settings: AttributesFormatString=<Deterministic=%<Deterministic>>
  Terminator : Terminator
  Transm_ECU : ModelReference  ModelNameDialog=TransmCtrl_V1_1.slx  SimulationMode=Normal  ModelReferenceVersion=1.0.41
  TransmCtrl : Outport
  tag scope: TransmCtrl_PwtrCAN_Tx=scoped
  wires:
  Transm_ECU/2 -> [TransmCtrl_PwtrCAN_Tx]  "TransmCtrl_PwtrCAN_Tx"
  Transm_ECU/1 -> Rate Transition5/1
  Rate Transition5/1 -> TransmCtrl/1  "TransmCtrl"
  Rate Transition3/1 -> Transm_ECU/1
  [TransmCtrl_PwtrCAN_Rx] -> Transm_ECU/3
  TM_sensor/1 -> Rate Transition4/1
  Driver_demand/1 -> Rate Transition3/1
  Transm_ECU/3 -> Terminator/1
  Rate Transition4/1 -> Transm_ECU/2

== system HEV_Simu_V1_1_RT/Controller/CtrlStrct_VNT_Level_2/VNT_Level_2_CAN/Battery_Ctrl ==
  note: Battery control
  note: CAN receive and transmit
  note: Battery Control
  PwtrCAN : Inport
  BatteryCtrl_PwtrCAN Tx : Subsystem
  BatteryCtrl_PwtrCAN_Rx : Subsystem
  BatteryCtrl_PwtrCAN_Tx : Outport
  tag scope: BatteryCtrl_PwtrCAN_Rx=scoped
  wires:
  [BatteryCtrl_PwtrCAN_Tx] -> BatteryCtrl_PwtrCAN Tx/1(BatteryCtrl_PwtrCAN_Tx_Apli)
  BatteryCtrl_PwtrCAN Tx/1(BatteryCtrl_PwtrCAN_Tx) -> BatteryCtrl_PwtrCAN_Tx/1
  PwtrCAN/1 -> BatteryCtrl_PwtrCAN_Rx/1(PwtrCAN)
  BatteryCtrl_PwtrCAN_Rx/1(BatteryCtrl_PwtrCAN_Rx) -> [BatteryCtrl_PwtrCAN_Rx]

== system HEV_Simu_V1_1_RT/Controller/CtrlStrct_VNT_Level_2/VNT_Level_2_CAN/Body_Ctrl ==
  note: Body Control
  note: CAN receive and transmit
  note: Body control
  VehCAN : Inport
  BodyCtrl_VehCAN Tx : Subsystem
  BodyCtrl_VehCAN_Rx : Subsystem
  BodyCtrl_VehCAN_Tx : Outport
  tag scope: BodyCtrl_VehCAN_Rx=scoped
  wires:
  [BodyCtrl_VehCAN_Tx] -> BodyCtrl_VehCAN Tx/1(BodyCtrl_VehCAN_Tx_Apli)
  BodyCtrl_VehCAN Tx/1(BodyCtrl_VehCAN_Tx) -> BodyCtrl_VehCAN_Tx/1
  VehCAN/1 -> BodyCtrl_VehCAN_Rx/1(VehCAN)
  BodyCtrl_VehCAN_Rx/1(BodyCtrl_VehCAN_Rx) -> [BodyCtrl_VehCAN_Rx]

== system HEV_Simu_V1_1_RT/Controller/CtrlStrct_VNT_Level_2/VNT_Level_2_CAN/Brake_Ctrl ==
  note: Brake Control
  note: CAN receive and transmit
  note: Brake control
  VehCAN : Inport
  BrakeCtrl_VehCAN Tx : Subsystem
  BrakeCtrl_VehCAN_Rx : Subsystem
  BrakeCtrl_VehCAN_Tx : Outport
  tag scope: BrakeCtrl_VehCAN_Rx=scoped
  wires:
  [BrakeCtrl_VehCAN_Tx] -> BrakeCtrl_VehCAN Tx/1(BrakeCtrl_VehCAN_Tx_Apli)
  BrakeCtrl_VehCAN Tx/1(BrakeCtrl_VehCAN_Tx) -> BrakeCtrl_VehCAN_Tx/1
  VehCAN/1 -> BrakeCtrl_VehCAN_Rx/1(VehCAN)
  BrakeCtrl_VehCAN_Rx/1(BrakeCtrl_VehCAN_Rx) -> [BrakeCtrl_VehCAN_Rx]

== system HEV_Simu_V1_1_RT/Controller/CtrlStrct_VNT_Level_2/VNT_Level_2_CAN/Engine_Ctrl ==
  note: Engine control
  note: Engine Control
  note: CAN receive and transmit
  PwtrCAN : Inport
  EngineCtrl_PwtrCAN Tx : Subsystem
  EngineCtrl_PwtrCAN_Rx : Subsystem
  EngineCtrl_PwtrCAN_Tx : Outport
  tag scope: EngineCtrl_PwtrCAN_Rx=scoped
  wires:
  [EngineCtrl_PwtrCAN_Tx] -> EngineCtrl_PwtrCAN Tx/1(EngineCtrl_PwtrCAN_Tx_Apli)
  EngineCtrl_PwtrCAN Tx/1(EngineCtrl_PwtrCAN_Tx) -> EngineCtrl_PwtrCAN_Tx/1
  PwtrCAN/1 -> EngineCtrl_PwtrCAN_Rx/1(PwtrCAN)
  EngineCtrl_PwtrCAN_Rx/1(EngineCtrl_PwtrCAN_Rx) -> [EngineCtrl_PwtrCAN_Rx]

== system HEV_Simu_V1_1_RT/Controller/CtrlStrct_VNT_Level_2/VNT_Level_2_CAN/Gateway ==
  note: Gateway
  InfoCAN : Inport
  VehCAN : Inport  Port=2
  PwtrCAN : Inport  Port=3
  Gateway InfoCAN : Subsystem
  Gateway PwtrCAN : Subsystem
  Gateway VehCAN : Subsystem
  Info Hub : Subsystem
  Gateway_PwtrCAN_Tx : Outport
  Gateway_VehCAN_Tx : Outport  Port=2
  Gateway_InfoCAN_Tx : Outport  Port=3
  wires:
  InfoCAN/1 -> Gateway PwtrCAN/1(InfoCAN), Info Hub/1(InfoCAN), Gateway VehCAN/1(InfoCAN)
  PwtrCAN/1 -> Info Hub/3(PwtrCAN), Gateway VehCAN/2(PwtrCAN)
  Gateway InfoCAN/1(Gateway_InfoCAN) -> Gateway_InfoCAN_Tx/1
  Gateway VehCAN/1(Gateway_VehCAN_Tx) -> Gateway_VehCAN_Tx/1
  Gateway PwtrCAN/1(Gateway_PwtrCAN_Tx) -> Gateway_PwtrCAN_Tx/1
  VehCAN/1 -> Gateway InfoCAN/1(VehCAN), Gateway PwtrCAN/2(VehCAN), Info Hub/2(VehCAN)
  Gateway PwtrCAN/2(VehSpd) -> Gateway InfoCAN/2(VehSpd)

== system HEV_Simu_V1_1_RT/Controller/CtrlStrct_VNT_Level_2/VNT_Level_2_CAN/HEV_Ctrl ==
  note: HEV control
  note: HEV control
  note: CAN receive and transmit
  PwtrCAN : Inport
  HEV_Ctrl_PwtrCAN Tx : Subsystem
  HEV_Ctrl_PwtrCAN_Rx : Subsystem
  HEV_Ctrl_PwtrCAN_Tx : Outport
  tag scope: HEV_Ctrl_PwtrCAN_Rx=scoped
  wires:
  [HEV_Ctrl_PwtrCAN_Tx] -> HEV_Ctrl_PwtrCAN Tx/1(HEV_Ctrl_PwtrCAN_Tx_Apli)
  HEV_Ctrl_PwtrCAN Tx/1(HEV_Ctrl_PwtrCAN_Tx) -> HEV_Ctrl_PwtrCAN_Tx/1
  PwtrCAN/1 -> HEV_Ctrl_PwtrCAN_Rx/1(PwtrCAN)
  HEV_Ctrl_PwtrCAN_Rx/1(HEV_Ctrl_PwtrCAN_Rx) -> [HEV_Ctrl_PwtrCAN_Rx]

== system HEV_Simu_V1_1_RT/Controller/CtrlStrct_VNT_Level_2/VNT_Level_2_CAN/HVAC_Ctrl ==
  note: HVAC control
  note: CAN receive and transmit
  note: HVAC Control
  VehCAN : Inport
  HVAC_Ctrl_VehCAN Tx : Subsystem
  HVAC_Ctrl_VehCAN_Rx : Subsystem
  HVAC_Ctrl_VehCAN_Tx : Outport
  tag scope: HVAC_Ctrl_VehCAN_Rx=scoped
  wires:
  [HVAC_Ctrl_VehCAN_Tx] -> HVAC_Ctrl_VehCAN Tx/1(HVAC_Ctrl_VehCAN_Tx_Apli)
  HVAC_Ctrl_VehCAN Tx/1(HVAC_Ctrl_VehCAN_Tx) -> HVAC_Ctrl_VehCAN_Tx/1
  VehCAN/1 -> HVAC_Ctrl_VehCAN_Rx/1(VehCAN)
  HVAC_Ctrl_VehCAN_Rx/1(HVAC_Ctrl_VehCAN_Rx) -> [HVAC_Ctrl_VehCAN_Rx]

== system HEV_Simu_V1_1_RT/Controller/CtrlStrct_VNT_Level_2/VNT_Level_2_CAN/InfoCAN ==
  note: Infotainment CAN
  Gateway_InfoCAN : Inport
  NAVI_InfoCAN_Tx : Inport  Port=2
  Radar_InfoCAN_Tx : Inport  Port=3
  Bus Creator : BusCreator  Inputs=3
  Bus Selector : BusSelector  OutputSignals=Gateway_InfoCAN_Tx_0CFFC485
  Bus Selector1 : BusSelector  OutputSignals=NAVI_InfoCAN_Tx_0CFFB01C
  Bus Selector2 : BusSelector  OutputSignals=Radar_InfoCAN_Tx_0CFF0080
  CAN_Memory : Memory
  InfoCAN : Outport
  wires:
  Bus Creator/1 -> CAN_Memory/1  "InfoCAN"
  Radar_InfoCAN_Tx/1 -> Bus Selector2/1
  CAN_Memory/1 -> InfoCAN/1  "InfoCAN"
  Gateway_InfoCAN/1 -> Bus Selector/1
  NAVI_InfoCAN_Tx/1 -> Bus Selector1/1
  Bus Selector/1 -> Bus Creator/1  "<Gateway_InfoCAN_Tx_0CFFC485>"
  Bus Selector1/1 -> Bus Creator/2  "<NAVI_InfoCAN_Tx_0CFFB01C>"
  Bus Selector2/1 -> Bus Creator/3  "<Radar_InfoCAN_Tx_0CFF0080>"

== system HEV_Simu_V1_1_RT/Controller/CtrlStrct_VNT_Level_2/VNT_Level_2_CAN/Motor_Ctrl ==
  note: Motor control
  note: Motor Control
  note: CAN receive and transmit
  PwtrCAN : Inport
  MotorCtrl_PwtrCAN Tx : Subsystem
  MotorCtrl_PwtrCAN_Rx : Subsystem
  MotorCtrl_PwtrCAN_Tx : Outport
  tag scope: MotorCtrl_PwtrCAN_Rx=scoped
  wires:
  [MotorCtrl_PwtrCAN_Tx] -> MotorCtrl_PwtrCAN Tx/1(IMotorCtrl_PwtrCAN_Tx_Apli)
  MotorCtrl_PwtrCAN Tx/1(MotorCtrl_PwtrCAN_Tx_0CFF5083) -> MotorCtrl_PwtrCAN_Tx/1
  PwtrCAN/1 -> MotorCtrl_PwtrCAN_Rx/1(PwtrCAN)
  MotorCtrl_PwtrCAN_Rx/1(MotorCtrl_PwtrCAN_Rx) -> [MotorCtrl_PwtrCAN_Rx]

== system HEV_Simu_V1_1_RT/Controller/CtrlStrct_VNT_Level_2/VNT_Level_2_CAN/NAVI ==
  note: Navigation
  note: CAN receive and transmit
  note: Navigation
  InfoCAN : Inport
  NAVI_CAN_Rx : Subsystem
  NAVI_CAN_Tx : Subsystem
  NAVI_InfoCAN_Tx : Outport
  tag scope: NAVI_InfoCAN_Rx=scoped
  wires:
  NAVI_CAN_Rx/1(NAVI_InfoCAN_Rx) -> [NAVI_InfoCAN_Rx]  "NAVI_InfoCAN_Rx"
  [NAVI_InfoCAN_Tx] -> NAVI_CAN_Tx/1(NAVI_InfoCAN_Tx_Apli)
  NAVI_CAN_Tx/1(NAVI_InfoCAN_Tx) -> NAVI_InfoCAN_Tx/1
  InfoCAN/1 -> NAVI_CAN_Rx/1(InfoCAN)

== system HEV_Simu_V1_1_RT/Controller/CtrlStrct_VNT_Level_2/VNT_Level_2_CAN/PwtrCAN ==
  Gateway_PwtrCAN_Tx : Inport
  HEV_Ctrl_PwtrCAN_Tx : Inport  Port=2
  EngineCtrl_PwtrCAN_Tx : Inport  Port=3
  TransmCtrl_PwtrCAN_Tx : Inport  Port=4
  MotorCtrl_PwtrCAN_Tx : Inport  Port=5
  BatteryCtrl_PwtrCAN_Tx : Inport  Port=6
  Bus Creator3 : BusCreator  Inputs=8
  Bus Selector : BusSelector  OutputSignals=Gateway_PwtrCAN_Tx_0CFFC285,Gateway_PwtrCAN_Tx_0CFFC385
  Bus Selector1 : BusSelector  OutputSignals=HEV_Ctrl_PwtrCAN_Tx_0CFF2082,HEV_Ctrl_PwtrCAN_Tx_0CFF2182
  Bus Selector2 : BusSelector  OutputSignals=BatteryCtrl_PwtrCAN_Tx_0CFF8084
  Bus Selector3 : BusSelector  OutputSignals=EngineCtrl_PwtrCAN_Tx_0CFF3000
  Bus Selector4 : BusSelector  OutputSignals=MotorCtrl_PwtrCAN_Tx_0CFF5083
  Bus Selector5 : BusSelector  OutputSignals=TransmCtrl_PwtrCAN_Tx_0CFF4003
  PwtrCAN_Memory : Memory
  PwtrCAN : Outport
  wires:
  TransmCtrl_PwtrCAN_Tx/1 -> Bus Selector5/1
  Bus Creator3/1 -> PwtrCAN_Memory/1  "PwtrCAN"
  EngineCtrl_PwtrCAN_Tx/1 -> Bus Selector3/1
  Gateway_PwtrCAN_Tx/1 -> Bus Selector/1
  HEV_Ctrl_PwtrCAN_Tx/1 -> Bus Selector1/1
  BatteryCtrl_PwtrCAN_Tx/1 -> Bus Selector2/1
  MotorCtrl_PwtrCAN_Tx/1 -> Bus Selector4/1
  PwtrCAN_Memory/1 -> PwtrCAN/1  "PwtrCAN"
  Bus Selector/1 -> Bus Creator3/1  "<Gateway_PwtrCAN_Tx_0CFFC285>"
  Bus Selector/2 -> Bus Creator3/2  "<Gateway_PwtrCAN_Tx_0CFFC385>"
  Bus Selector1/1 -> Bus Creator3/3  "<HEV_Ctrl_PwtrCAN_Tx_0CFF2082>"
  Bus Selector1/2 -> Bus Creator3/4  "<HEV_Ctrl_PwtrCAN_Tx_0CFF2182>"
  Bus Selector2/1 -> Bus Creator3/8  "<BatteryCtrl_PwtrCAN_Tx_0CFF8084>"
  Bus Selector3/1 -> Bus Creator3/5  "<EngineCtrl_PwtrCAN_Tx_0CFF3000>"
  Bus Selector4/1 -> Bus Creator3/7  "<MotorCtrl_PwtrCAN_Tx_0CFF5083>"
  Bus Selector5/1 -> Bus Creator3/6  "<TransmCtrl_PwtrCAN_Tx_0CFF4003>"

== system HEV_Simu_V1_1_RT/Controller/CtrlStrct_VNT_Level_2/VNT_Level_2_CAN/Radar ==
  note: Radar detection
  note: CAN receive and transmit
  note: Radar Detection
  InfoCAN : Inport
  Radar_CAN_Rx : Subsystem
  Radar_CAN_Tx : Subsystem
  Radar_InfoCAN_Tx : Outport
  tag scope: Radar_InfoCAN_Rx=scoped
  wires:
  [Radar_InfoCAN_Tx] -> Radar_CAN_Tx/1(Radar_InfoCAN_Tx_Apli)
  Radar_CAN_Tx/1(Radar_InfoCAN_Tx) -> Radar_InfoCAN_Tx/1
  Radar_CAN_Rx/1(Radar_InfoCAN_Rx) -> [Radar_InfoCAN_Rx]
  InfoCAN/1 -> Radar_CAN_Rx/1(InfoCAN)

== system HEV_Simu_V1_1_RT/Controller/CtrlStrct_VNT_Level_2/VNT_Level_2_CAN/Steer_Ctrl ==
  note: Steering control
  note: CAN receive and transmit
  note: Steering Control
  VehCAN : Inport
  SteerCtrl_VehCAN Tx : Subsystem
  SteerCtrl_VehCAN_Rx : Subsystem
  SteerCtrl_VehCAN_Tx : Outport
  tag scope: SteerCtrl_VehCAN_Rx=scoped
  wires:
  [SteerCtrl_VehCAN_Tx] -> SteerCtrl_VehCAN Tx/1(SteerCtrl_VehCAN_Tx_Apli)
  SteerCtrl_VehCAN Tx/1(SteerCtrl_VehCAN_Tx) -> SteerCtrl_VehCAN_Tx/1
  VehCAN/1 -> SteerCtrl_VehCAN_Rx/1(In1)
  SteerCtrl_VehCAN_Rx/1(SteerCtrl_VehCAN_Rx) -> [SteerCtrl_VehCAN_Rx]

== system HEV_Simu_V1_1_RT/Controller/CtrlStrct_VNT_Level_2/VNT_Level_2_CAN/Transms_Ctrl ==
  note: Transmission control
  note: CAN receive and transmit
  note: Transmission Control
  PwtrCAN : Inport
  TransmCtrl_PwtrCAN Tx : Subsystem
  TransmCtrl_PwtrCAN_Rx : Subsystem
  TransmCtrl_PwtrCAN_Tx : Outport
  tag scope: TransmCtrl_PwtrCAN_Rx=scoped
  wires:
  [TransmCtrl_PwtrCAN_Tx] -> TransmCtrl_PwtrCAN Tx/1(TransmCtrl_PwtrCAN_Tx_Apli)
  TransmCtrl_PwtrCAN Tx/1(TransmCtrl_PwtrCAN_Tx) -> TransmCtrl_PwtrCAN_Tx/1
  PwtrCAN/1 -> TransmCtrl_PwtrCAN_Rx/1(PwtrCAN)
  TransmCtrl_PwtrCAN_Rx/1(TransmCtrl_PwtrCAN_Rx) -> [TransmCtrl_PwtrCAN_Rx]

== system HEV_Simu_V1_1_RT/Controller/CtrlStrct_VNT_Level_2/VNT_Level_2_CAN/VM_Ctrl ==
  note: Vehicle motion control
  note: Vehicle Motion Control
  note: CAN receive and transmit
  VehCAN : Inport
  VM_Ctrl_VehCAN Tx : Subsystem
  VM_Ctrl_VehCAN_Rx : Subsystem
  VM_Ctrl_VehCAN_Tx : Outport
  tag scope: VM_Ctrl_VehCAN_Rx=scoped
  wires:
  [VM_Ctrl_VehCAN_Tx] -> VM_Ctrl_VehCAN Tx/1(VM_Ctrl_VehCAN_Tx_Apli)
  VM_Ctrl_VehCAN Tx/1(VM_Ctrl_VehCAN_Tx) -> VM_Ctrl_VehCAN_Tx/1
  VehCAN/1 -> VM_Ctrl_VehCAN_Rx/1(In1)
  VM_Ctrl_VehCAN_Rx/1(VM_Ctrl_VehCAN_Rx) -> [VM_Ctrl_VehCAN_Rx]

== system HEV_Simu_V1_1_RT/Controller/CtrlStrct_VNT_Level_2/VNT_Level_2_CAN/VehCAN ==
  note: Vehicle CAN
  Gateway_VehCAN_Tx : Inport
  VM_Ctrl_VehCAN_Tx : Inport  Port=2
  BrakeCtrl_VehCAN_Tx : Inport  Port=3
  SteerCtrl_VehCAN_Tx : Inport  Port=4
  HVAC_Ctrl_VehCAN_Tx : Inport  Port=5
  BodyCtrl_VehCAN_Tx : Inport  Port=6
  Bus Creator1 : BusCreator  Inputs=7
  Bus Selector : BusSelector  OutputSignals=Gateway_VehCAN_Tx_0CFFC085,Gateway_VehCAN_Tx_0CFFC185
  Bus Selector1 : BusSelector  OutputSignals=BodyCtrl_VehCAN_Tx_0CFFA028
  Bus Selector2 : BusSelector  OutputSignals=BrakeCtrl_VehCAN_Tx_0CFF600B
  Bus Selector3 : BusSelector  OutputSignals=HVAC_Ctrl_VehCAN_Tx_0CFFE087
  Bus Selector4 : BusSelector  OutputSignals=SteerCtrl_VehCAN_Tx_0CFF7013
  Bus Selector5 : BusSelector  OutputSignals=VM_Ctrl_VehCAN_Tx_0CFFD086
  VehCAN_Memory : Memory
  VehCAN : Outport
  wires:
  VehCAN_Memory/1 -> VehCAN/1  "VehCAN"
  SteerCtrl_VehCAN_Tx/1 -> Bus Selector4/1
  BrakeCtrl_VehCAN_Tx/1 -> Bus Selector2/1
  Gateway_VehCAN_Tx/1 -> Bus Selector/1
  Bus Creator1/1 -> VehCAN_Memory/1  "VehCAN"
  BodyCtrl_VehCAN_Tx/1 -> Bus Selector1/1
  HVAC_Ctrl_VehCAN_Tx/1 -> Bus Selector3/1
  VM_Ctrl_VehCAN_Tx/1 -> Bus Selector5/1
  Bus Selector/1 -> Bus Creator1/1  "<Gateway_VehCAN_Tx_0CFFC085>"
  Bus Selector/2 -> Bus Creator1/2  "<Gateway_VehCAN_Tx_0CFFC185>"
  Bus Selector1/1 -> Bus Creator1/7  "<BodyCtrl_VehCAN_Tx_0CFFA028>"
  Bus Selector2/1 -> Bus Creator1/4  "<BrakeCtrl_VehCAN_Tx_0CFF600B>"
  Bus Selector3/1 -> Bus Creator1/6  "<HVAC_Ctrl_VehCAN_Tx_0CFFE087>"
  Bus Selector4/1 -> Bus Creator1/5  "<SteerCtrl_VehCAN_Tx_0CFF7013>"
  Bus Selector5/1 -> Bus Creator1/3  "<VM_Ctrl_VehCAN_Tx_0CFFD086>"

== system HEV_Simu_V1_1_RT/Controller/CtrlStrct_VNT_Level_2/Vehicle/HEV_Control ==
  note: HEV Control
  Driver_demand : Inport
  HEV_sensor : Inport  Port=2
  HEV_Control : ModelReference  ModelNameDialog=HEV_Ctrl_V1_1.slx  SimulationMode=Normal  ModelReferenceVersion=1.0.51
  Rate Transition2 : RateTransition  Deterministic=off
      settings: AttributesFormatString=<Deterministic=%<Deterministic>>
  Rate Transition3 : RateTransition  Deterministic=off
      settings: AttributesFormatString=<Deterministic=%<Deterministic>>
  Rate Transition4 : RateTransition  Deterministic=off
      settings: AttributesFormatString=<Deterministic=%<Deterministic>>
  tag scope: HEV_Ctrl_PwtrCAN_Tx=scoped, HEV_ECU_Info=global
  wires:
  Rate Transition3/1 -> HEV_Control/1
  HEV_Control/1 -> [HEV_Ctrl_PwtrCAN_Tx]  "HEV_Ctrl_PwtrCAN_Tx"
  Rate Transition4/1 -> [HEV_ECU_Info]  "HEV_Ctrl_Info"
  HEV_Control/2 -> Rate Transition4/1
  Rate Transition2/1 -> HEV_Control/2
  HEV_sensor/1 -> Rate Transition2/1
  [HEV_Ctrl_PwtrCAN_Rx] -> HEV_Control/3
  Driver_demand/1 -> Rate Transition3/1
